simulink model "requirements01_backup"  (R2024a)
settings: Solver=VariableStepAuto  StartTime=0.0  StopTime=10.0  RelTol=1e-3
settings Model: Creator=amir  LastModifiedBy=amir

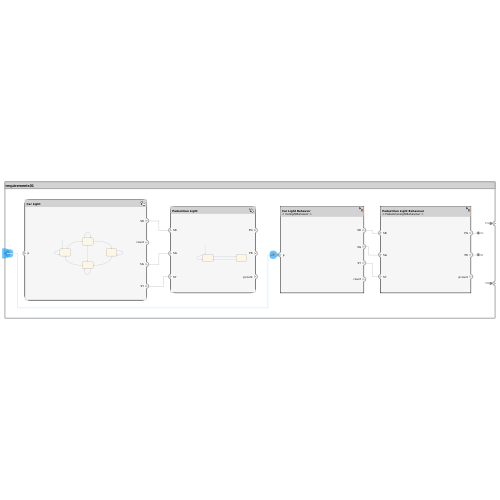
[thumbnail: Simulink's stored preview of the top-level diagram]
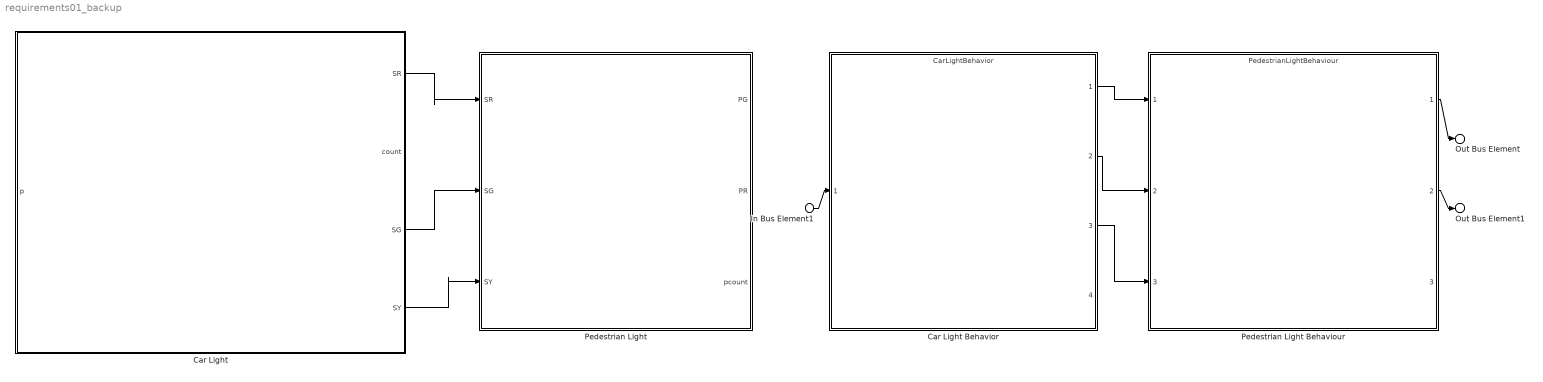
== system requirements01_backup ==
  In Bus Element1 : Inport  PortName=p
  Car Light : Stateflow chart  TreatAsAtomicUnit=on
      settings: PortSchema="{\"entries\":[{\"content\":{\"headerSize\":26,\"margin\":15,\"minimumSpacing\":25,\"sides\":[{\"content\":{\"connectorIds\":[\"In1\"]},\"type\":\"ConnectorPlacement.EquallySpacedRectSide\",\"uuid\":\"dcad2c70-2645-4f1a-8a68-18ec1ad8ba87\"},{\"content\":{\"connectorIds\":[\"Out1\",\"Out2\",\"Out3\",\"Out4\"],\"side\":\"RIGHT\"},\"type\":\"ConnectorPlacement.EquallySpacedRectSide\",\"uuid\":\"d956afcc-b59b-4cd9-bf0c-2faf54410a1f\"},{\"content\":{\"side\":\"TOP\"},\"type\":\"ConnectorPlacement.EquallySpacedRectSide\",\"uuid\":\"630f687d-dbcb-4c68-a5cf-c443c2c2bd85\"},{\"content\":{\"side\":\"BOTTOM\"},\"type\":\"ConnectorPlacement.EquallySpacedRectSide\",\"uuid\":\"3a3e5d4a-5477-4627-aecc-2fafaa003a9f\"}]},\"type\":\"ConnectorPlacement.EquallySpacedConnector\",\"uuid\":\"08b6b339-ecb4-42d5-aaa8-85a19f994eb0\"}],\"packageUris\":[\"http://schema.mathworks.com/mf0/Connector/R2020b\"],\"version\":\"1.0\"}"
  Car Light Behavior : ModelReference  ModelNameDialog=CarLightBehavior  SimulationMode=Normal  ModelReferenceVersion=1.2
      settings: PortSchema="{\"entries\":[{\"content\":{\"headerSize\":38,\"margin\":15,\"minimumSpacing\":25,\"sides\":[{\"content\":{\"connectorIds\":[\"In1\"]},\"type\":\"ConnectorPlacement.EquallySpacedRectSide\",\"uuid\":\"48726829-d86d-461c-b3f1-a9b4bbd6b695\"},{\"content\":{\"connectorIds\":[\"Out1\",\"Out2\",\"Out3\",\"Out4\"],\"side\":\"RIGHT\"},\"type\":\"ConnectorPlacement.EquallySpacedRectSide\",\"uuid\":\"4ff77f49-fdf8-4120-97ad-bb22e2b131c5\"},{\"content\":{\"side\":\"TOP\"},\"type\":\"ConnectorPlacement.EquallySpacedRectSide\",\"uuid\":\"b9798bfe-0ecf-4d40-a284-8acf4e1ad550\"}]},\"type\":\"ConnectorPlacement.EquallySpacedConnector\",\"uuid\":\"dfbb9b41-0bc8-4650-9c2d-4ffd36c28d79\"}],\"packageUris\":[\"http://schema.mathworks.com/mf0/Connector/R2020b\"],\"version\":\"1.0\"}"
  Pedestrian Light : Stateflow chart  TreatAsAtomicUnit=on
      settings: PortSchema="{\"entries\":[{\"content\":{\"headerSize\":26,\"margin\":15,\"minimumSpacing\":25,\"sides\":[{\"content\":{\"connectorIds\":[\"In1\",\"In2\",\"In3\"]},\"type\":\"ConnectorPlacement.EquallySpacedRectSide\",\"uuid\":\"dcad2c70-2645-4f1a-8a68-18ec1ad8ba87\"},{\"content\":{\"connectorIds\":[\"Out1\",\"Out2\",\"Out3\"],\"side\":\"RIGHT\"},\"type\":\"ConnectorPlacement.EquallySpacedRectSide\",\"uuid\":\"d956afcc-b59b-4cd9-bf0c-2faf54410a1f\"},{\"content\":{\"side\":\"TOP\"},\"type\":\"ConnectorPlacement.EquallySpacedRectSide\",\"uuid\":\"630f687d-dbcb-4c68-a5cf-c443c2c2bd85\"}]},\"type\":\"ConnectorPlacement.EquallySpacedConnector\",\"uuid\":\"08b6b339-ecb4-42d5-aaa8-85a19f994eb0\"}],\"packageUris\":[\"http://schema.mathworks.com/mf0/Connector/R2020b\"],\"version\":\"1.0\"}"
  Pedestrian Light Behaviour : ModelReference  ModelNameDialog=PedestrianLightBehaviour  SimulationMode=Normal  ModelReferenceVersion=1.2
      settings: PortSchema="{\"entries\":[{\"content\":{\"headerSize\":38,\"margin\":15,\"minimumSpacing\":25,\"sides\":[{\"content\":{\"connectorIds\":[\"In1\",\"In2\",\"In3\"]},\"type\":\"ConnectorPlacement.EquallySpacedRectSide\",\"uuid\":\"48726829-d86d-461c-b3f1-a9b4bbd6b695\"},{\"content\":{\"connectorIds\":[\"Out1\",\"Out2\",\"Out3\"],\"side\":\"RIGHT\"},\"type\":\"ConnectorPlacement.EquallySpacedRectSide\",\"uuid\":\"4ff77f49-fdf8-4120-97ad-bb22e2b131c5\"},{\"content\":{\"side\":\"TOP\"},\"type\":\"ConnectorPlacement.EquallySpacedRectSide\",\"uuid\":\"b9798bfe-0ecf-4d40-a284-8acf4e1ad550\"}]},\"type\":\"ConnectorPlacement.EquallySpacedConnector\",\"uuid\":\"dfbb9b41-0bc8-4650-9c2d-4ffd36c28d79\"}],\"packageUris\":[\"http://schema.mathworks.com/mf0/Connector/R2020b\"],\"version\":\"1.0\"}"
  Out Bus Element : Outport  PortName=PG
  Out Bus Element1 : Outport  Port=2  PortName=PR
  wires:
  Car Light/1(SR) -> Pedestrian Light/1(SR)
  Car Light/3(SG) -> Pedestrian Light/2(SG)
  Car Light/4(SY) -> Pedestrian Light/3(SY)
  Car Light Behavior/1 -> Pedestrian Light Behaviour/1
  Car Light Behavior/2 -> Pedestrian Light Behaviour/2
  Car Light Behavior/3 -> Pedestrian Light Behaviour/3
  Pedestrian Light Behaviour/1 -> Out Bus Element/1
  Pedestrian Light Behaviour/2 -> Out Bus Element1/1
  In Bus Element1/1 -> Car Light Behavior/1

== stateflow chart requirements01_backup/Car Light ==
  state Green
  state Red
  state Yellow
  state Pending
  Green -> Green [order 1] : [count<60]{count=count+1; SG=0;}
  (default) -> Red : {count=0;}
  Red -> Green [order 1] : [count>=60]{SG=1; SR=0; count=0;}
  Green -> Yellow [order 2] : [p==1 && count<60]{SG=0;}
  Green -> Pending [order 3] : [p==1 && count>=60]{SG=0; SY=1; count=0;}
  Yellow -> Yellow [order 2] : {count=count+1}
  Red -> Red [order 2] : {count=count+1; SR=0;}
  Pending -> Red [order 1] : [count>=5]{SR=1; count=0;}
  Yellow -> Pending [order 1] : [count>=60]{SY=1; count=0;}
  Pending -> Pending [order 2] : {count=count+1; SY=0}
  data: p input; SR output; count output; SG output; SY output

== stateflow chart requirements01_backup/Pedestrian Light ==
  state green
  state red
  (default) -> green : {pcount=0;}
  green -> green [order 2] : {pcount=pcount+1; PG=0}
  green -> red [order 1] : [pcount>=55]{PR=1; PG=0}
  red -> green : [SR]{pcount=0; PG=1; PR=0}
  data: SR input; PG output; PR output; pcount output; SG input; SY input
